simulink model "jacobian_inverse"  (R2019b)
settings: Solver=VariableStepAuto  StartTime=0.0  StopTime=4.0  RelTol=1e-3
undefined symbols (not defined in the file): DiscIntNeverNeededParam, q0, Tc
settings Model: Creator=rajath  LastModifiedBy=GA

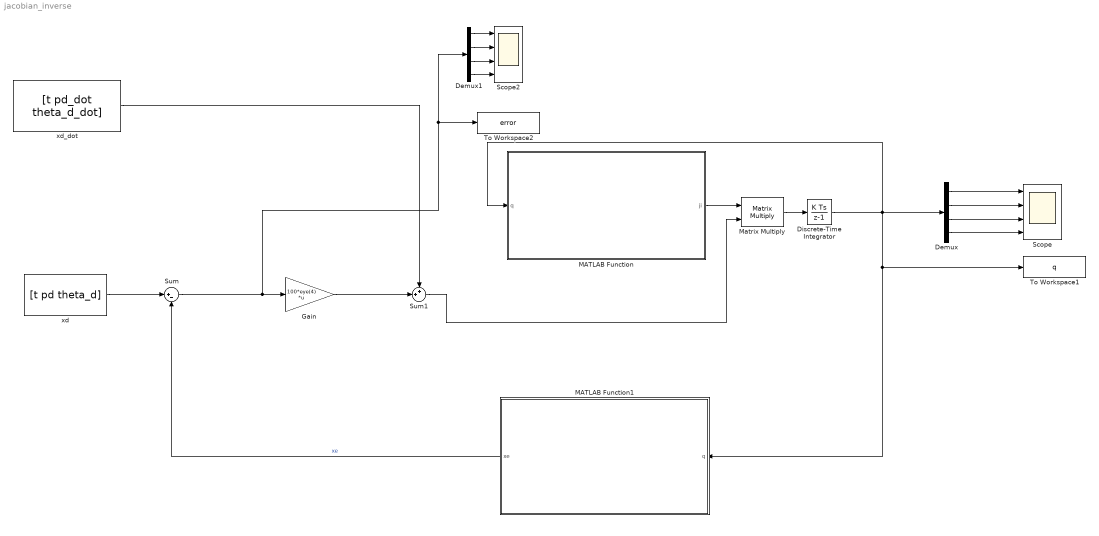
== system jacobian_inverse ==
  Demux : Demux
  Demux1 : Demux
  Discrete-Time Integrator : DiscreteIntegrator  gainval=1  InitialCondition=q0  SampleTime=Tc  ICPrevOutput=DiscIntNeverNeededParam  ICPrevScaledInput=DiscIntNeverNeededParam
  Gain : Gain  Gain=100*eye(4)  Multiplication=Matrix(K*u)
  MATLAB Function : MATLAB Function  TreatAsAtomicUnit=on
  MATLAB Function1 : MATLAB Function  TreatAsAtomicUnit=on
  Matrix Multiply : Product  Multiplication=Matrix(*)
  Scope : Scope  NumInputPorts=4
  Scope2 : Scope  NumInputPorts=4
  Sum : Sum  Inputs=|+-
  Sum1 : Sum  Inputs=++|
  To Workspace1 : ToWorkspace  VariableName=q  SaveFormat=Timeseries  SampleTime=-1
  To Workspace2 : ToWorkspace  VariableName=error  SaveFormat=Timeseries  SampleTime=Tc
  xd : FromWorkspace  VariableName=[t pd theta_d]  SampleTime=Tc
  xd_dot : FromWorkspace  VariableName=[t pd_dot theta_d_dot]  SampleTime=Tc
  wires:
  xd/1 -> Sum/1
  Sum/1 -> To Workspace2/1, Demux1/1, Gain/1
  xd_dot/1 -> Sum1/1
  Discrete-Time Integrator/1 -> MATLAB Function/1(q), Demux/1, MATLAB Function1/1(q), To Workspace1/1
  MATLAB Function1/1(xe) -> Sum/2  "xe"
  MATLAB Function/1(ji) -> Matrix Multiply/1
  Matrix Multiply/1 -> Discrete-Time Integrator/1
  Gain/1 -> Sum1/2
  Sum1/1 -> Matrix Multiply/2
  Demux/3 -> Scope/3
  Demux/2 -> Scope/2
  Demux/1 -> Scope/1
  Demux/4 -> Scope/4
  Demux1/1 -> Scope2/1
  Demux1/2 -> Scope2/2
  Demux1/3 -> Scope2/3
  Demux1/4 -> Scope2/4

== matlab function jacobian_inverse/MATLAB Function1 ==
  data: q input; xe output
function xe = non_linear_function(q)
a1 = 0.5;
a2 = 0.5;
d0 = 1;
xe = zeros(4,1);
xe(1,:) = a1*cos(q(1))+a2*cos(q(1)+q(2));
xe(2,:) = a1*sin(q(1))+a2*sin(q(1)+q(2));
xe(3,:) = d0 - q(3);
xe(4,:) = (q(1)+q(2)+q(4));

== matlab function jacobian_inverse/MATLAB Function ==
  data: q input; ji output
function ji = jacobian_inverse(q)
    
a1 = 0.5;
a2 = 0.5;

j = zeros(4,4);
j(1,1) = -a1*sin(q(1))-a2*sin(q(1)+q(2));
j(1,2) = -a2*sin(q(1)+q(2));
j(2,1) = a1*cos(q(1))+a2*cos(q(1)+q(2));
j(2,2) = a2*cos(q(1)+q(2));
j(3,3) = -1;
j(4,1) = 1;
j(4,2) = 1;
j(4,4) = 1;
ji = j'*inv(j*j');
